simulink model "ABS_off"  (R2020b)
settings: Solver=VariableStepAuto  StartTime=0.0  StopTime=60.0  RelTol=1e-3
InitFcn:
  | lam_opt = [
  |            0.17
  |            0.13
  |            0.16
  |            0.14
  |            0.06
  |            0.03
  |           ];
values from neighbouring files (symbols this model uses):
  ce = road_coeff(sel,:)    [ABS_ga.m]    (also in ABS_pso.m)
  g = 9.81    [ABS_ga.m]    (also in ABS_pso.m)
  J = 1.13    [ABS_ga.m]    (also in ABS_pso.m)
  PID = [ ... (first row only)    [road_anfis.m]
  T_B = 0.1    [ABS_ga.m]    (also in ABS_pso.m)
undefined symbols (not defined in the file or in its folder): m, R, sel, v_x
libraries: pid_lib x1
settings Model: Creator=hadlaczkyb  LastModifiedBy=hadlaczkyb
settings DataIOCC: ReturnWorkspaceOutputs=off
settings DebuggingCC: ArithmeticOperatorsInVariantConditions=warning
settings SFSimCC: SimUseLocalCustomCode=off  CustomCodeUndefinedFunction=UseInterfaceOnly
settings RTWCC: RTWUseLocalCustomCode=off

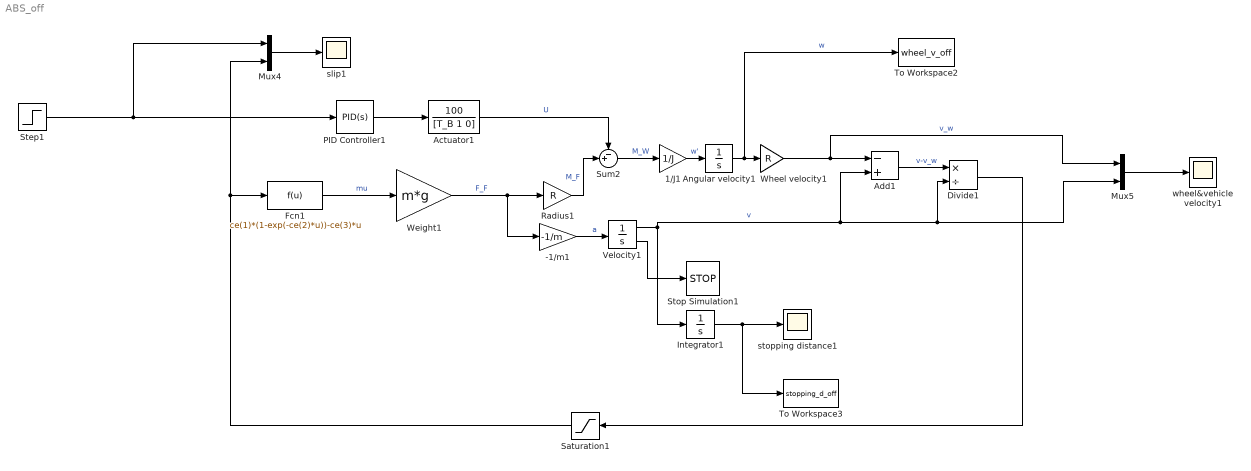
== system ABS_off ==
  -1/m1 : Gain  Gain=-1/m
  1/J1 : Gain  Gain=1/J
  Actuator1 : TransferFcn  Numerator=[0 0 100]  Denominator=[T_B 1 0]
  Add1 : Sum  Inputs=-+
  Angular velocity1 : Integrator  InitialCondition=v_x/R  LimitOutput=on  UpperSaturationLimit=1000  LowerSaturationLimit=0
  Divide1 : Product  Inputs=*/
  Fcn1 : Fcn  Expr=ce(1)*(1-exp(-ce(2)*u))-ce(3)*u
  Integrator1 : Integrator
  Mux4 : Mux  Inputs=2
  Mux5 : Mux  Inputs=2
  PID Controller1 : pid_lib/PID Controller  Controller=PID  Form=Parallel  TimeDomain=Continuous-time  UseExternalTs=off  SampleTime=-1  IntegratorMethod=Forward Euler  FilterMethod=Forward Euler  ControllerParametersSource=internal  P=PID(sel,1)  I=PID(sel,2)  D=PID(sel,3)  UseFilter=on  N=1000  TunerSelectOption=Transfer Function Based (PID Tuner App)  InitialConditionSource=internal  InitialConditionForIntegrator=0  InitialConditionForFilter=0  DifferentiatorICPrevScaledInput=0  ExternalReset=none  TrackingMode=off  Kt=1  LimitOutput=off  SatLimitsSource=internal  UpperSaturationLimit=inf  LowerSaturationLimit=-inf  LinearizeAsGain=on  AntiWindupMode=none  Kb=1  POutMin=[]  POutMax=[]  IOutMin=[]  IOutMax=[]  DOutMin=[]  DOutMax=[]  NOutMin=[]  NOutMax=[]  SumOutMin=[]  SumOutMax=[]  SaturationOutMin=[]  SaturationOutMax=[]  PParamMin=[]  PParamMax=[]  IParamMin=[]  IParamMax=[]  DParamMin=[]  DParamMax=[]  NParamMin=[]  NParamMax=[]  KbParamMin=[]  KbParamMax=[]  KtParamMin=[]  KtParamMax=[]  KbOutMin=[]  KbOutMax=[]  KtOutMin=[]  KtOutMax=[]  IntegratorOutMin=[]  IntegratorOutMax=[]  FilterOutMin=[]  FilterOutMax=[]  SumI1OutMin=[]  SumI1OutMax=[]  SumI2OutMin=[]  SumI2OutMax=[]  SumI3OutMin=[]  SumI3OutMax=[]  SumI4OutMin=[]  SumI4OutMax=[]  SumDOutMin=[]  SumDOutMax=[]  DifferentiatorOutMin=[]  DifferentiatorOutMax=[]  FilterDiffOutCoefMin=[]  FilterDiffOutCoefMax=[]  ReciprocalOutMin=[]  ReciprocalOutMax=[]  SumDenOutMin=[]  SumDenOutMax=[]  SumNumOutMin=[]  SumNumOutMax=[]  DivideOutMin=[]  DivideOutMax=[]  UdiffTsProdOutMin=[]  UdiffTsProdOutMax=[]  NTsProdOutMin=[]  NTsProdOutMax=[]  UintegralTsProdOutMin=[]  UintegralTsProdOutMax=[]  UngainTsProdOutMin=[]  UngainTsProdOutMax=[]  IntegratorContinuousStateAttributes=''  IntegratorStateMustResolveToSignalObject=off  IntegratorRTWStateStorageClass=Auto  FilterContinuousStateAttributes=''  FilterStateMustResolveToSignalObject=off  FilterRTWStateStorageClass=Auto  ParallelPVariant=InternalParameters  IdealPVariant=Disabled  IVariant=InternalParameters  DVariant=InternalParameters  IntegratorVariant=Continuous  SatVariant=Disabled  AWVariant=Passthrough  PCopyVariant=Disabled  TRVariant=Disabled  FdbkBlocksVariant=Forward  IdealPFdbkVariant=Disabled  SatFdbkVariant=Disabled  DerivativeFilterVariant=ContFilter  NVariant=InternalParameters  NCopyVariant=Disabled  FilterICVariant=InternalICsFilter  IntegratorICVariant=InternalICs  ExternalResetVariant=Disabled  TRSumVariant=Passthrough  SumFdbkVariant=Disabled  SumVariant=Sum_PID  TsampFilterVariant=InternalTs  TsampNgainVariant=Passthrough  TsampIntegralVariant=Passthrough  ExternalSaturationOutDataTypeStr=Inherit: Same as second input
  Radius1 : Gain  Gain=R
  Saturation1 : Saturate  UpperLimit=1  LowerLimit=0
  Step1 : Step  Time=5  After=lam_opt(sel)  SampleTime=0
  Stop Simulation1 : Stop
  Sum2 : Sum  Inputs=-+|
  To Workspace2 : ToWorkspace  VariableName=wheel_v_off  SaveFormat=Timeseries  SampleTime=-1
  To Workspace3 : ToWorkspace  VariableName=stopping_d_off  SaveFormat=Timeseries  SampleTime=-1
  Velocity1 : Integrator  InitialCondition=v_x  LimitOutput=on  UpperSaturationLimit=1000  LowerSaturationLimit=1  ShowSaturationPort=on
  Weight1 : Gain  Gain=m*g
  Wheel velocity1 : Gain  Gain=R
  slip1 : Scope
  stopping distance1 : Scope
  wheel&vehicle velocity1 : Scope
  wires:
  Step1/1 -> PID Controller1/1, Mux4/1
  PID Controller1/1 -> Actuator1/1
  Mux4/1 -> slip1/1
  Radius1/1 -> Sum2/2  "M_F"
  Actuator1/1 -> Sum2/1  "U"
  Saturation1/1 -> Fcn1/1, Mux4/2
  Divide1/1 -> Saturation1/1
  1/J1/1 -> Angular velocity1/1  "w'"
  -1/m1/1 -> Velocity1/1  "a"
  Fcn1/1 -> Weight1/1  "mu"
  Wheel velocity1/1 -> Add1/1, Mux5/1  "v_w"
  Velocity1/2 -> Stop Simulation1/1
  Sum2/1 -> 1/J1/1  "M_W"
  Integrator1/1 -> To Workspace3/1, stopping distance1/1
  Mux5/1 -> wheel&vehicle velocity1/1
  Angular velocity1/1 -> To Workspace2/1, Wheel velocity1/1  "w"
  Velocity1/1 -> Integrator1/1, Add1/2, Divide1/2, Mux5/2  "v"
  Weight1/1 -> -1/m1/1, Radius1/1  "F_F"
  Add1/1 -> Divide1/1  "v-v_w"
